simulink library "Near1p1Ann"  (R2022b)
settings: Solver=VariableStepAuto  StartTime=0.0  StopTime=10.0  RelTol=1e-3
libraries: Upmixer1p1Lib x3, FeaturePath x2, FsEQLib x2, HrEQLib x2, Router x2, HandyTextFile x1, TuneVar x1, NearBandSplitLib x1, VolumeMute x1
settings Model: Creator=ak1044356  LastModifiedBy=sa1045272
settings SolverCC: AlgebraicLoopSolver=TrustRegion
settings DebuggingCC: UnconnectedInputMsg=warning  UnconnectedOutputMsg=warning  UnconnectedLineMsg=warning  SFMachineParentedDataDiag=warning  ArithmeticOperatorsInVariantConditions=warning
settings ModelReferenceCC: EnableRefExpFcnMdlSchedulingChecks=on
settings SFSimCC: CustomCodeUndefinedFunction=UseInterfaceOnly

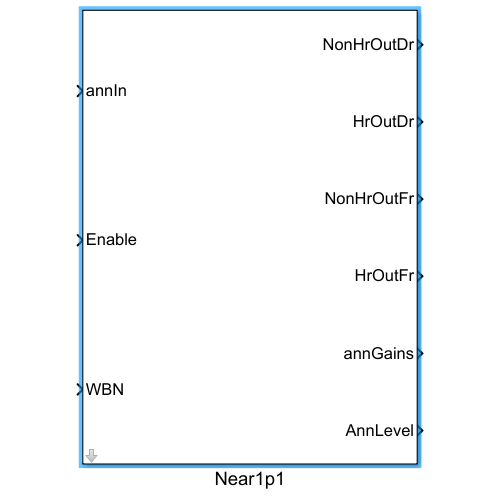
[thumbnail: Simulink's stored preview of the top-level diagram]
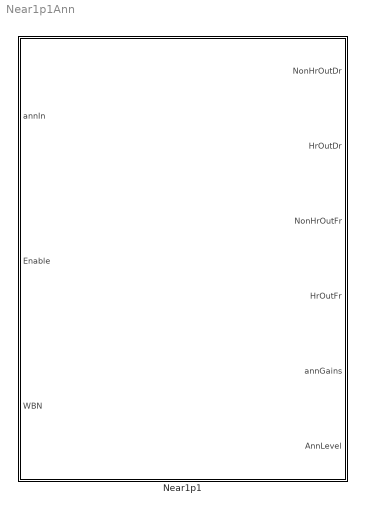
== system Near1p1Ann ==
  Near1p1 : Subsystem  mask{Config=[]}
      mask prompts: Config "Near1p1Config"
      mask init:
      | blkh=gcbh;
      | Config=BTConfig.Assert(blkh,Config);
      | % sample_rate_in_hertz                        = near.sample_rate_in_hertz;
      | % frame_size                                  = near.frame_size;
      | % ann_sysin_channel_count                     = near.ann_sysin_channel_count;
      | % front_peripheral_channel_count              = near.front_peripheral_channel_count;
      | % NEAR1p1FrontPeripheralChannelCountFullRate  = near.NEAR1p1FrontPeripheralChannelCountFullRate;
      | % NearWbAnnCount                              = near.NearWbAnnCount;
      | % headrest_count                              = near.headrest_count;
      | % channels_per_headrest                       = near.channels_per_headrest;
      | % decimation_factor                           = near.decimation_factor;
      | % rear_channel_count                          = near.rear_channel_count;
      | % vm                                          = near.vm;
      | % decimated_frame_size                        = near.decimated_frame_size;
      | % decimated_sample_rate_in_hertz              = near.decimated_sample_rate_in_hertz;
      | Config.Validate();
      | Config.DoMaskInit(blkh);

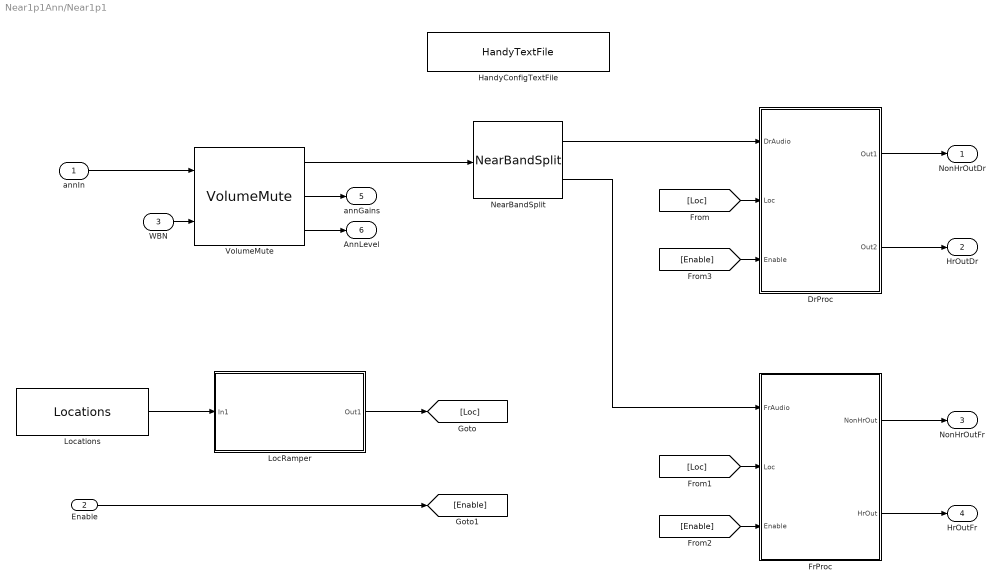
== system Near1p1Ann/Near1p1 ==
  annIn : Inport  OutDataTypeStr=single
  Enable : Inport  Port=2
  WBN : Inport  Port=3
  DrProc : Subsystem
  FrProc : Subsystem
  HandyConfigTextFile : HandyTextFile/HandyTextFile  TemplateSource=Config  FileSuffix=File  OpenDialogOnLoad=off  UseThisBlockName=off  AddGrandParentNamePrefix=off  TheDefaultText=% $(FILENAME) $(PREFIX) $(SUFFIX)  ShowInLibBrowser=on
      settings: SourceProductName=Bose Talaria
  LocRamper : Subsystem
  Locations : Upmixer1p1Lib/Locations  SystemSampleTime=-1  VariantActivationTime=update diagram  Latency=0  AutoFrameSizeCalculation=off
  NearBandSplit : NearBandSplitLib/NearBandSplit  Config=Config.NearBandSplit
  VolumeMute : VolumeMute/VolumeMute  Config=Config.VolumeMute
  NonHrOutDr : Outport  VectorParamsAs1DForOutWhenUnconnected=off
  HrOutDr : Outport  Port=2  VectorParamsAs1DForOutWhenUnconnected=off
  NonHrOutFr : Outport  Port=3  VectorParamsAs1DForOutWhenUnconnected=off
  HrOutFr : Outport  Port=4  VectorParamsAs1DForOutWhenUnconnected=off
  annGains : Outport  Port=5
  AnnLevel : Outport  Port=6
  wires:
  annIn/1 -> VolumeMute/1
  VolumeMute/1 -> NearBandSplit/1
  VolumeMute/2 -> annGains/1
  WBN/1 -> VolumeMute/2
  VolumeMute/3 -> AnnLevel/1
  NearBandSplit/1 -> DrProc/1(DrAudio)
  DrProc/1(Out1) -> NonHrOutDr/1
  DrProc/2(Out2) -> HrOutDr/1
  NearBandSplit/2 -> FrProc/1(FrAudio)
  FrProc/1(NonHrOut) -> NonHrOutFr/1
  FrProc/2(HrOut) -> HrOutFr/1
  Enable/1 -> [Enable]
  Locations/1 -> LocRamper/1(In1)
  [Loc] -> DrProc/2(Loc)
  [Loc] -> FrProc/2(Loc)
  [Enable] -> FrProc/3(Enable)
  [Enable] -> DrProc/3(Enable)
  LocRamper/1(Out1) -> [Loc]

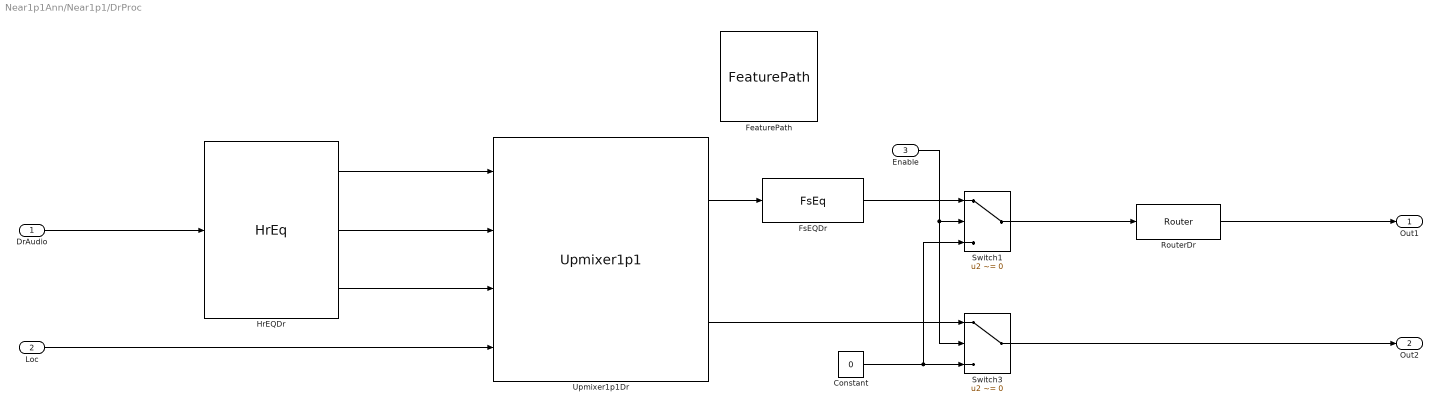
== system Near1p1Ann/Near1p1/DrProc ==
  DrAudio : Inport
  Loc : Inport  Port=2
  Enable : Inport  Port=3
  Constant : Constant  Value=0  OutDataTypeStr=single
  FeaturePath : FeaturePath/FeaturePath  FeatureName=Dr_  IsGroup=off  GroupNumber=-1  IsModule=off  TriggerInit=[730 -106 845 1]
      settings: SourceProductName=Bose Talaria
  FsEQDr : FsEQLib/FsEq  Config=Config.FsEqDr
  HrEQDr : HrEQLib/HrEq  Config=Config.HrEqDr
  RouterDr : Router/Router  nInRouterMask=Config.NearRouterNumIn  nOutRouterMask=Config.NearRouterNumOut  outputMapDefaultRouterMask=Config.NearRouterMap
  Switch1 : Switch  Criteria=u2 ~= 0  Threshold=.5  ZeroCross=off  SaturateOnIntegerOverflow=off  InputSameDT=off
  Switch3 : Switch  Criteria=u2 ~= 0  Threshold=.5  ZeroCross=off  SaturateOnIntegerOverflow=off  InputSameDT=off
  Upmixer1p1Dr : Upmixer1p1Lib/Upmixer1p1  Config=Config.Upmixer1p1Dr
  Out1 : Outport
  Out2 : Outport  Port=2
  wires:
  Switch1/1 -> RouterDr/1
  Constant/1 -> Switch1/3, Switch3/3
  RouterDr/1 -> Out1/1
  FsEQDr/1 -> Switch1/1
  Switch3/1 -> Out2/1
  Enable/1 -> Switch3/2, Switch1/2
  Loc/1 -> Upmixer1p1Dr/4
  DrAudio/1 -> HrEQDr/1
  Upmixer1p1Dr/2 -> Switch3/1
  Upmixer1p1Dr/1 -> FsEQDr/1
  HrEQDr/3 -> Upmixer1p1Dr/3
  HrEQDr/1 -> Upmixer1p1Dr/1
  HrEQDr/2 -> Upmixer1p1Dr/2

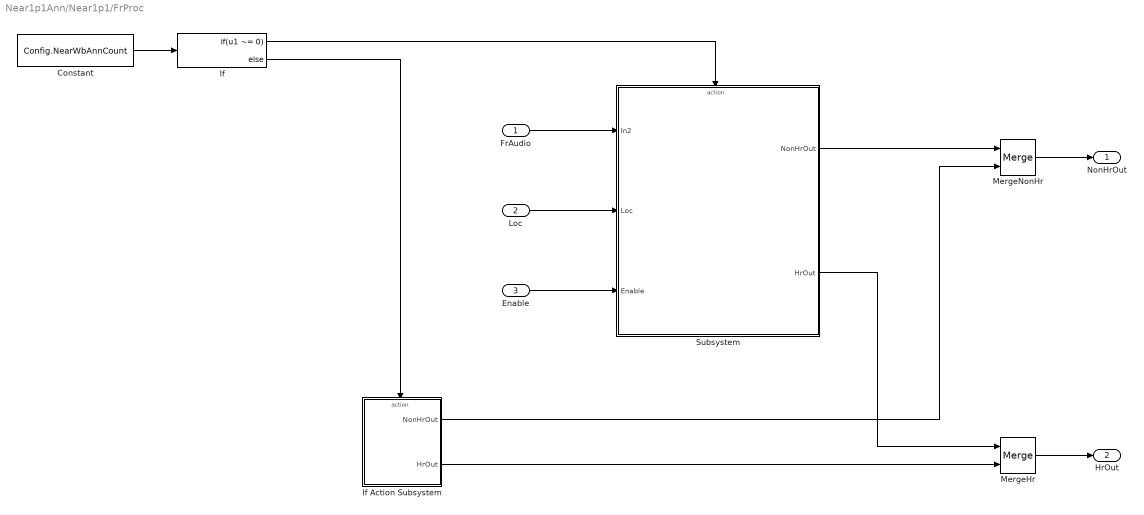
== system Near1p1Ann/Near1p1/FrProc ==
  FrAudio : Inport
  Loc : Inport  Port=2
  Enable : Inport  Port=3
  Constant : Constant  Value=Config.NearWbAnnCount
  If : If  IfExpression=u1 ~= 0
  If Action Subsystem : Subsystem  TreatAsAtomicUnit=on
  MergeHr : Merge
  MergeNonHr : Merge
  Subsystem : Subsystem
  NonHrOut : Outport
  HrOut : Outport  Port=2
  wires:
  Enable/1 -> Subsystem/3(Enable)
  FrAudio/1 -> Subsystem/1(In2)
  Loc/1 -> Subsystem/2(Loc)
  Subsystem/1(NonHrOut) -> MergeNonHr/1
  Subsystem/2(HrOut) -> MergeHr/1
  If/1 -> Subsystem/Action
  If/2 -> If Action Subsystem/Action
  MergeHr/1 -> HrOut/1
  MergeNonHr/1 -> NonHrOut/1
  If Action Subsystem/1(NonHrOut) -> MergeNonHr/2
  If Action Subsystem/2(HrOut) -> MergeHr/2
  Constant/1 -> If/1

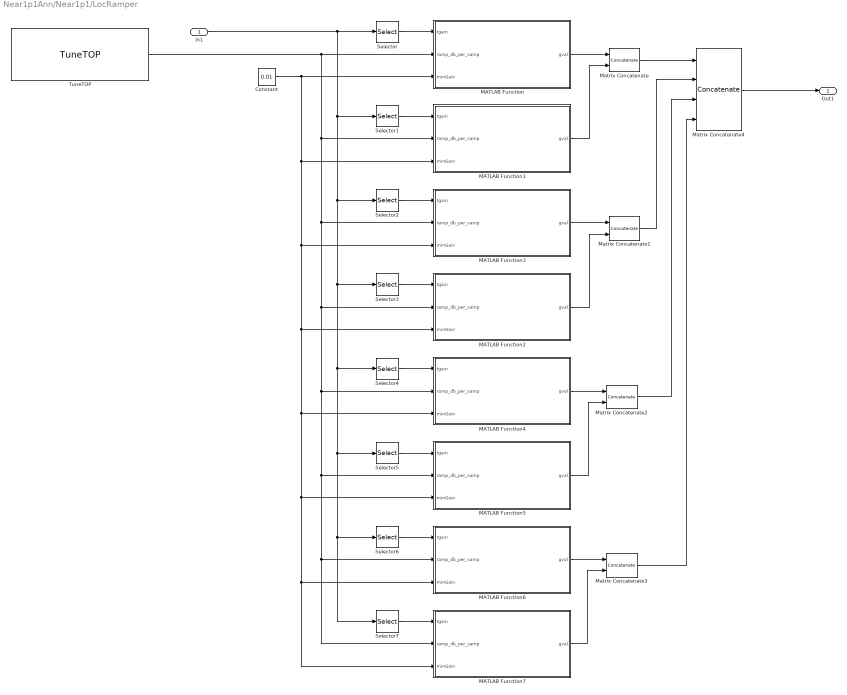
== system Near1p1Ann/Near1p1/LocRamper ==
  In1 : Inport
  Constant : Constant  Value=0.01
  MATLAB Function : MATLAB Function  TreatAsAtomicUnit=on  mask{FRAME_SIZE=Config.FrameSize}
  MATLAB Function1 : MATLAB Function  TreatAsAtomicUnit=on  mask{FRAME_SIZE=Config.FrameSize}
  MATLAB Function2 : MATLAB Function  TreatAsAtomicUnit=on  mask{FRAME_SIZE=Config.FrameSize}
  MATLAB Function3 : MATLAB Function  TreatAsAtomicUnit=on  mask{FRAME_SIZE=Config.FrameSize}
  MATLAB Function4 : MATLAB Function  TreatAsAtomicUnit=on  mask{FRAME_SIZE=Config.FrameSize}
  MATLAB Function5 : MATLAB Function  TreatAsAtomicUnit=on  mask{FRAME_SIZE=Config.FrameSize}
  MATLAB Function6 : MATLAB Function  TreatAsAtomicUnit=on  mask{FRAME_SIZE=Config.FrameSize}
  MATLAB Function7 : MATLAB Function  TreatAsAtomicUnit=on  mask{FRAME_SIZE=Config.FrameSize}
  Matrix Concatenate{,1..3} (4 alike) : Concatenate  Mode=Multidimensional array
  Matrix Concatenate4 : Concatenate  NumInputs=4  Mode=Multidimensional array  ConcatenateDimension=3
  Selector : Selector  NumberOfDimensions=3  InputPortWidth=3  IndexOptions=Index vector (dialog),Index vector (dialog),Index vector (dialog)  Indices=1,1,1  OutputSizes=1,1,1
  Selector1 : Selector  NumberOfDimensions=3  InputPortWidth=3  IndexOptions=Index vector (dialog),Index vector (dialog),Index vector (dialog)  Indices=2,1,1  OutputSizes=1,1,1
  Selector2 : Selector  NumberOfDimensions=3  InputPortWidth=3  IndexOptions=Index vector (dialog),Index vector (dialog),Index vector (dialog)  Indices=1,1,2  OutputSizes=1,1,1
  Selector3 : Selector  NumberOfDimensions=3  InputPortWidth=3  IndexOptions=Index vector (dialog),Index vector (dialog),Index vector (dialog)  Indices=2,1,2  OutputSizes=1,1,1
  Selector4 : Selector  NumberOfDimensions=3  InputPortWidth=3  IndexOptions=Index vector (dialog),Index vector (dialog),Index vector (dialog)  Indices=1,1,3  OutputSizes=1,1,1
  Selector5 : Selector  NumberOfDimensions=3  InputPortWidth=3  IndexOptions=Index vector (dialog),Index vector (dialog),Index vector (dialog)  Indices=2,1,3  OutputSizes=1,1,1
  Selector6 : Selector  NumberOfDimensions=3  InputPortWidth=3  IndexOptions=Index vector (dialog),Index vector (dialog),Index vector (dialog)  Indices=1,1,4  OutputSizes=1,1,1
  Selector7 : Selector  NumberOfDimensions=3  InputPortWidth=3  IndexOptions=Index vector (dialog),Index vector (dialog),Index vector (dialog)  Indices=2,1,4  OutputSizes=1,1,1
  TuneTOP : TuneVar/TuneTOP  TriggerInit=[-300 49 -55 141]  TopName=RampDbPerSample  TuneName=RampDbPerSample  DataType=single  TunabilityNumber=1  MinValue=[]  MaxValue=[]  BankNumber=0  PreOverlay=false  PostOverlay=false  UseSameName=on  MaskValue=Config.DefaultRampDbPerSample
      settings: SourceProductName=Bose Talaria
  Out1 : Outport
  wires:
  Selector/1 -> MATLAB Function/1(tgain)
  TuneTOP/1 -> MATLAB Function7/2(ramp_db_per_samp), MATLAB Function6/2(ramp_db_per_samp), MATLAB Function5/2(ramp_db_per_samp), MATLAB Function4/2(ramp_db_per_samp), MATLAB Function2/2(ramp_db_per_samp), MATLAB Function3/2(ramp_db_per_samp), MATLAB Function1/2(ramp_db_per_samp), MATLAB Function/2(ramp_db_per_samp)
  Matrix Concatenate1/1 -> Matrix Concatenate4/2
  MATLAB Function2/1(gval) -> Matrix Concatenate1/2
  In1/1 -> Selector7/1, Selector6/1, Selector5/1, Selector4/1, Selector3/1, Selector2/1, Selector1/1, Selector/1
  Matrix Concatenate/1 -> Matrix Concatenate4/1
  Selector7/1 -> MATLAB Function7/1(tgain)
  MATLAB Function/1(gval) -> Matrix Concatenate/1
  Selector2/1 -> MATLAB Function3/1(tgain)
  Selector5/1 -> MATLAB Function5/1(tgain)
  MATLAB Function4/1(gval) -> Matrix Concatenate2/1
  Selector1/1 -> MATLAB Function1/1(tgain)
  Selector3/1 -> MATLAB Function2/1(tgain)
  MATLAB Function6/1(gval) -> Matrix Concatenate3/1
  Matrix Concatenate2/1 -> Matrix Concatenate4/3
  MATLAB Function1/1(gval) -> Matrix Concatenate/2
  Selector6/1 -> MATLAB Function6/1(tgain)
  Matrix Concatenate4/1 -> Out1/1
  MATLAB Function7/1(gval) -> Matrix Concatenate3/2
  Matrix Concatenate3/1 -> Matrix Concatenate4/4
  Selector4/1 -> MATLAB Function4/1(tgain)
  MATLAB Function5/1(gval) -> Matrix Concatenate2/2
  MATLAB Function3/1(gval) -> Matrix Concatenate1/1
  Constant/1 -> MATLAB Function7/3(minGain), MATLAB Function6/3(minGain), MATLAB Function5/3(minGain), MATLAB Function4/3(minGain), MATLAB Function2/3(minGain), MATLAB Function3/3(minGain), MATLAB Function1/3(minGain), MATLAB Function/3(minGain)

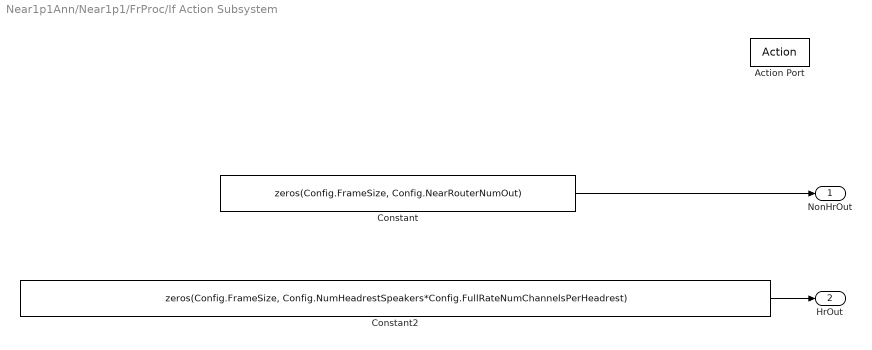
== system Near1p1Ann/Near1p1/FrProc/If Action Subsystem ==
  Action Port : ActionPort  ActionPortLabel=else
  Constant : Constant  Value=zeros(Config.FrameSize, Config.NearRouterNumOut)  OutDataTypeStr=single
  Constant2 : Constant  Value=zeros(Config.FrameSize, Config.NumHeadrestSpeakers*Config.FullRateNumChannelsPerHeadrest)  OutDataTypeStr=single
  NonHrOut : Outport
  HrOut : Outport  Port=2
  wires:
  Constant/1 -> NonHrOut/1
  Constant2/1 -> HrOut/1

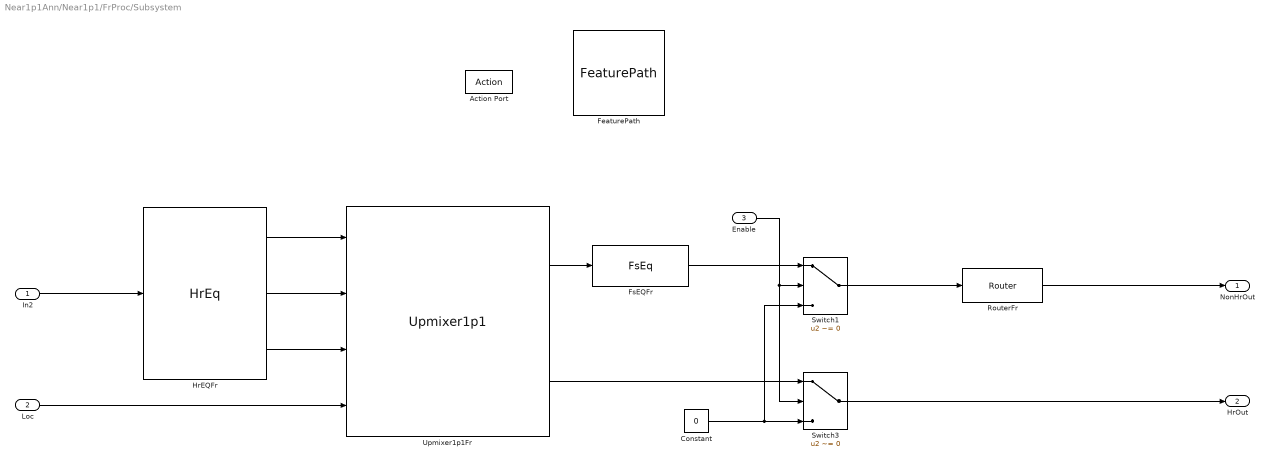
== system Near1p1Ann/Near1p1/FrProc/Subsystem ==
  In2 : Inport
  Loc : Inport  Port=2
  Enable : Inport  Port=3
  Action Port : ActionPort  PropagateVarSize=During execution  ActionPortLabel=if(u1 ~= 0)
  Constant : Constant  Value=0  OutDataTypeStr=single
  FeaturePath : FeaturePath/FeaturePath  FeatureName=Fr_  IsGroup=off  GroupNumber=-1  IsModule=off  TriggerInit=[760 79 875 186]
      settings: SourceProductName=Bose Talaria
  FsEQFr : FsEQLib/FsEq  Config=Config.FsEqFr
  HrEQFr : HrEQLib/HrEq  Config=Config.HrEqFr
  RouterFr : Router/Router  nInRouterMask=Config.NearRouterNumIn  nOutRouterMask=Config.NearRouterNumOut  outputMapDefaultRouterMask=Config.NearRouterMap
  Switch1 : Switch  Criteria=u2 ~= 0  Threshold=.5  ZeroCross=off  SaturateOnIntegerOverflow=off  InputSameDT=off
  Switch3 : Switch  Criteria=u2 ~= 0  Threshold=.5  ZeroCross=off  SaturateOnIntegerOverflow=off  InputSameDT=off
  Upmixer1p1Fr : Upmixer1p1Lib/Upmixer1p1  Config=Config.Upmixer1p1Fr
  NonHrOut : Outport
  HrOut : Outport  Port=2
  wires:
  FsEQFr/1 -> Switch1/1
  Constant/1 -> Switch1/3, Switch3/3
  In2/1 -> HrEQFr/1
  Switch1/1 -> RouterFr/1
  Enable/1 -> Switch3/2, Switch1/2
  RouterFr/1 -> NonHrOut/1
  Switch3/1 -> HrOut/1
  Upmixer1p1Fr/1 -> FsEQFr/1
  Upmixer1p1Fr/2 -> Switch3/1
  Loc/1 -> Upmixer1p1Fr/4
  HrEQFr/3 -> Upmixer1p1Fr/3
  HrEQFr/2 -> Upmixer1p1Fr/2
  HrEQFr/1 -> Upmixer1p1Fr/1

== matlab function Near1p1Ann/Near1p1/LocRamper/MATLAB Function ==
  data: tgain input; gval output; ramp_db_per_samp input; minGain input; FRAME_SIZE parameter
function gval = ramp(tgain, ramp_db_per_samp, minGain, FRAME_SIZE)
% FRAME_SIZE = 32;
% Ramp coefficients
persistent lastTGain;
if (isempty(lastTGain)), lastTGain = cast(tgain + 1, class(tgain)); end
persistent lastG;
if (isempty(lastG)), lastG = cast(0, class(tgain)); end
% Ramp coefficients
persistent upCoeff;
if (isempty(upCoeff)), upCoeff = cast(0, class(tgain)); end
persistent upCoeffN;
if (isempty(upCoeffN)), upCoeffN = cast(0, class(tgain)); end
persistent downCoeff;
if (isempty(downCoeff)), downCoeff = cast(0, class(tgain)); end
persistent downCoeffN;
if (isempty(downCoeffN)), downCoeffN = cast(0, class(tgain)); end
persistent nextUpCoeff;
persistent nextUpCoeffN;
persistent nextDownCoeff;
persistent nextDownCoeffN;
persistent lpfCoeff;
if (isempty(lpfCoeff)), lpfCoeff = cast(exp(-1 / FRAME_SIZE), class(tgain)); end
% Update the next set of ramp coefficients to use
nextUpCoeff = cast(10 ^ abs(ramp_db_per_samp / 20), class(tgain));
nextUpCoeffN = cast(nextUpCoeff ^ FRAME_SIZE, class(tgain));
nextDownCoeff = cast(10 ^ (-abs(ramp_db_per_samp) / 20), class(tgain));
nextDownCoeffN = cast(nextDownCoeff ^ FRAME_SIZE, class(tgain));
% Switch to the next set of ramp coefficients if the target gain changed
chtgain = (tgain ~= lastTGain);
lastTGain = tgain;
if (chtgain)
    upCoeff = nextUpCoeff;
    upCoeffN = nextUpCoeffN;
    downCoeff = nextDownCoeff;
    downCoeffN = nextDownCoeffN;
end
% Initialize output
gp = lastG;
gdiff = tgain - gp;
% By default, use the lpf filter
a = lpfCoeff;
b0 = 1-a;

if (abs(gdiff) < minGain)
    % Snap to target gain if it's close enough
    gVec = tgain * ones(FRAME_SIZE, 1, class(tgain));
else
    if (gdiff > 0)
        % previous gain cannot be zero for exponential ramp
        temp = max(gp, minGain);
        if (temp * upCoeffN < tgain)
            % Ramp not done, so do zero-input exponential ramp
            a = upCoeff;
            b0 = cast(0, class(tgain));
            gp = temp;
        end
    else
        if (gp * downCoeffN > tgain)
            % Ramp not done, so do zero-input exponential ramp
            a = downCoeff;
            b0 = cast(0, class(tgain));
        end
    end
    % Calculate gain
    zi = a * gp;
    gVec = zeros(FRAME_SIZE, 1, class(tgain));
    for samp = 1:FRAME_SIZE
        g = b0 * tgain + zi;
        zi = a * g;
        gVec(samp) = g;
    end
end
lastG = gVec(end);
gval = lastG;
end

== matlab function Near1p1Ann/Near1p1/LocRamper/MATLAB Function1 ==
  data: tgain input; gval output; ramp_db_per_samp input; minGain input; FRAME_SIZE parameter
function gval = ramp(tgain, ramp_db_per_samp, minGain, FRAME_SIZE)
% FRAME_SIZE = 32;
% Ramp coefficients
persistent lastTGain;
if (isempty(lastTGain)), lastTGain = cast(tgain + 1, class(tgain)); end
persistent lastG;
if (isempty(lastG)), lastG = cast(0, class(tgain)); end
% Ramp coefficients
persistent upCoeff;
if (isempty(upCoeff)), upCoeff = cast(0, class(tgain)); end
persistent upCoeffN;
if (isempty(upCoeffN)), upCoeffN = cast(0, class(tgain)); end
persistent downCoeff;
if (isempty(downCoeff)), downCoeff = cast(0, class(tgain)); end
persistent downCoeffN;
if (isempty(downCoeffN)), downCoeffN = cast(0, class(tgain)); end
persistent nextUpCoeff;
persistent nextUpCoeffN;
persistent nextDownCoeff;
persistent nextDownCoeffN;
persistent lpfCoeff;
if (isempty(lpfCoeff)), lpfCoeff = cast(exp(-1 / FRAME_SIZE), class(tgain)); end
% Update the next set of ramp coefficients to use
nextUpCoeff = cast(10 ^ abs(ramp_db_per_samp / 20), class(tgain));
nextUpCoeffN = cast(nextUpCoeff ^ FRAME_SIZE, class(tgain));
nextDownCoeff = cast(10 ^ (-abs(ramp_db_per_samp) / 20), class(tgain));
nextDownCoeffN = cast(nextDownCoeff ^ FRAME_SIZE, class(tgain));
% Switch to the next set of ramp coefficients if the target gain changed
chtgain = (tgain ~= lastTGain);
lastTGain = tgain;
if (chtgain)
    upCoeff = nextUpCoeff;
    upCoeffN = nextUpCoeffN;
    downCoeff = nextDownCoeff;
    downCoeffN = nextDownCoeffN;
end
% Initialize output
gp = lastG;
gdiff = tgain - gp;
% By default, use the lpf filter
a = lpfCoeff;
b0 = 1-a;

if (abs(gdiff) < minGain)
    % Snap to target gain if it's close enough
    gVec = tgain * ones(FRAME_SIZE, 1, class(tgain));
else
    if (gdiff > 0)
        % previous gain cannot be zero for exponential ramp
        temp = max(gp, minGain);
        if (temp * upCoeffN < tgain)
            % Ramp not done, so do zero-input exponential ramp
            a = upCoeff;
            b0 = cast(0, class(tgain));
            gp = temp;
        end
    else
        if (gp * downCoeffN > tgain)
            % Ramp not done, so do zero-input exponential ramp
            a = downCoeff;
            b0 = cast(0, class(tgain));
        end
    end
    % Calculate gain
    zi = a * gp;
    gVec = zeros(FRAME_SIZE, 1, class(tgain));
    for samp = 1:FRAME_SIZE
        g = b0 * tgain + zi;
        zi = a * g;
        gVec(samp) = g;
    end
end
lastG = gVec(end);
gval = lastG;
end

== matlab function Near1p1Ann/Near1p1/LocRamper/MATLAB Function2 ==
  data: tgain input; gval output; ramp_db_per_samp input; minGain input; FRAME_SIZE parameter
function gval = ramp(tgain, ramp_db_per_samp, minGain, FRAME_SIZE)
% FRAME_SIZE = 32;
% Ramp coefficients
persistent lastTGain;
if (isempty(lastTGain)), lastTGain = cast(tgain + 1, class(tgain)); end
persistent lastG;
if (isempty(lastG)), lastG = cast(0, class(tgain)); end
% Ramp coefficients
persistent upCoeff;
if (isempty(upCoeff)), upCoeff = cast(0, class(tgain)); end
persistent upCoeffN;
if (isempty(upCoeffN)), upCoeffN = cast(0, class(tgain)); end
persistent downCoeff;
if (isempty(downCoeff)), downCoeff = cast(0, class(tgain)); end
persistent downCoeffN;
if (isempty(downCoeffN)), downCoeffN = cast(0, class(tgain)); end
persistent nextUpCoeff;
persistent nextUpCoeffN;
persistent nextDownCoeff;
persistent nextDownCoeffN;
persistent lpfCoeff;
if (isempty(lpfCoeff)), lpfCoeff = cast(exp(-1 / FRAME_SIZE), class(tgain)); end
% Update the next set of ramp coefficients to use
nextUpCoeff = cast(10 ^ abs(ramp_db_per_samp / 20), class(tgain));
nextUpCoeffN = cast(nextUpCoeff ^ FRAME_SIZE, class(tgain));
nextDownCoeff = cast(10 ^ (-abs(ramp_db_per_samp) / 20), class(tgain));
nextDownCoeffN = cast(nextDownCoeff ^ FRAME_SIZE, class(tgain));
% Switch to the next set of ramp coefficients if the target gain changed
chtgain = (tgain ~= lastTGain);
lastTGain = tgain;
if (chtgain)
    upCoeff = nextUpCoeff;
    upCoeffN = nextUpCoeffN;
    downCoeff = nextDownCoeff;
    downCoeffN = nextDownCoeffN;
end
% Initialize output
gp = lastG;
gdiff = tgain - gp;
% By default, use the lpf filter
a = lpfCoeff;
b0 = 1-a;

if (abs(gdiff) < minGain)
    % Snap to target gain if it's close enough
    gVec = tgain * ones(FRAME_SIZE, 1, class(tgain));
else
    if (gdiff > 0)
        % previous gain cannot be zero for exponential ramp
        temp = max(gp, minGain);
        if (temp * upCoeffN < tgain)
            % Ramp not done, so do zero-input exponential ramp
            a = upCoeff;
            b0 = cast(0, class(tgain));
            gp = temp;
        end
    else
        if (gp * downCoeffN > tgain)
            % Ramp not done, so do zero-input exponential ramp
            a = downCoeff;
            b0 = cast(0, class(tgain));
        end
    end
    % Calculate gain
    zi = a * gp;
    gVec = zeros(FRAME_SIZE, 1, class(tgain));
    for samp = 1:FRAME_SIZE
        g = b0 * tgain + zi;
        zi = a * g;
        gVec(samp) = g;
    end
end
lastG = gVec(end);
gval = lastG;
end

== matlab function Near1p1Ann/Near1p1/LocRamper/MATLAB Function3 ==
  data: tgain input; gval output; ramp_db_per_samp input; minGain input; FRAME_SIZE parameter
function gval = ramp(tgain, ramp_db_per_samp, minGain, FRAME_SIZE)
% FRAME_SIZE = 32;
% Ramp coefficients
persistent lastTGain;
if (isempty(lastTGain)), lastTGain = cast(tgain + 1, class(tgain)); end
persistent lastG;
if (isempty(lastG)), lastG = cast(0, class(tgain)); end
% Ramp coefficients
persistent upCoeff;
if (isempty(upCoeff)), upCoeff = cast(0, class(tgain)); end
persistent upCoeffN;
if (isempty(upCoeffN)), upCoeffN = cast(0, class(tgain)); end
persistent downCoeff;
if (isempty(downCoeff)), downCoeff = cast(0, class(tgain)); end
persistent downCoeffN;
if (isempty(downCoeffN)), downCoeffN = cast(0, class(tgain)); end
persistent nextUpCoeff;
persistent nextUpCoeffN;
persistent nextDownCoeff;
persistent nextDownCoeffN;
persistent lpfCoeff;
if (isempty(lpfCoeff)), lpfCoeff = cast(exp(-1 / FRAME_SIZE), class(tgain)); end
% Update the next set of ramp coefficients to use
nextUpCoeff = cast(10 ^ abs(ramp_db_per_samp / 20), class(tgain));
nextUpCoeffN = cast(nextUpCoeff ^ FRAME_SIZE, class(tgain));
nextDownCoeff = cast(10 ^ (-abs(ramp_db_per_samp) / 20), class(tgain));
nextDownCoeffN = cast(nextDownCoeff ^ FRAME_SIZE, class(tgain));
% Switch to the next set of ramp coefficients if the target gain changed
chtgain = (tgain ~= lastTGain);
lastTGain = tgain;
if (chtgain)
    upCoeff = nextUpCoeff;
    upCoeffN = nextUpCoeffN;
    downCoeff = nextDownCoeff;
    downCoeffN = nextDownCoeffN;
end
% Initialize output
gp = lastG;
gdiff = tgain - gp;
% By default, use the lpf filter
a = lpfCoeff;
b0 = 1-a;

if (abs(gdiff) < minGain)
    % Snap to target gain if it's close enough
    gVec = tgain * ones(FRAME_SIZE, 1, class(tgain));
else
    if (gdiff > 0)
        % previous gain cannot be zero for exponential ramp
        temp = max(gp, minGain);
        if (temp * upCoeffN < tgain)
            % Ramp not done, so do zero-input exponential ramp
            a = upCoeff;
            b0 = cast(0, class(tgain));
            gp = temp;
        end
    else
        if (gp * downCoeffN > tgain)
            % Ramp not done, so do zero-input exponential ramp
            a = downCoeff;
            b0 = cast(0, class(tgain));
        end
    end
    % Calculate gain
    zi = a * gp;
    gVec = zeros(FRAME_SIZE, 1, class(tgain));
    for samp = 1:FRAME_SIZE
        g = b0 * tgain + zi;
        zi = a * g;
        gVec(samp) = g;
    end
end
lastG = gVec(end);
gval = lastG;
end

== matlab function Near1p1Ann/Near1p1/LocRamper/MATLAB Function4 ==
  data: tgain input; gval output; ramp_db_per_samp input; minGain input; FRAME_SIZE parameter
function gval = ramp(tgain, ramp_db_per_samp, minGain, FRAME_SIZE)
% FRAME_SIZE = 32;
% Ramp coefficients
persistent lastTGain;
if (isempty(lastTGain)), lastTGain = cast(tgain + 1, class(tgain)); end
persistent lastG;
if (isempty(lastG)), lastG = cast(0, class(tgain)); end
% Ramp coefficients
persistent upCoeff;
if (isempty(upCoeff)), upCoeff = cast(0, class(tgain)); end
persistent upCoeffN;
if (isempty(upCoeffN)), upCoeffN = cast(0, class(tgain)); end
persistent downCoeff;
if (isempty(downCoeff)), downCoeff = cast(0, class(tgain)); end
persistent downCoeffN;
if (isempty(downCoeffN)), downCoeffN = cast(0, class(tgain)); end
persistent nextUpCoeff;
persistent nextUpCoeffN;
persistent nextDownCoeff;
persistent nextDownCoeffN;
persistent lpfCoeff;
if (isempty(lpfCoeff)), lpfCoeff = cast(exp(-1 / FRAME_SIZE), class(tgain)); end
% Update the next set of ramp coefficients to use
nextUpCoeff = cast(10 ^ abs(ramp_db_per_samp / 20), class(tgain));
nextUpCoeffN = cast(nextUpCoeff ^ FRAME_SIZE, class(tgain));
nextDownCoeff = cast(10 ^ (-abs(ramp_db_per_samp) / 20), class(tgain));
nextDownCoeffN = cast(nextDownCoeff ^ FRAME_SIZE, class(tgain));
% Switch to the next set of ramp coefficients if the target gain changed
chtgain = (tgain ~= lastTGain);
lastTGain = tgain;
if (chtgain)
    upCoeff = nextUpCoeff;
    upCoeffN = nextUpCoeffN;
    downCoeff = nextDownCoeff;
    downCoeffN = nextDownCoeffN;
end
% Initialize output
gp = lastG;
gdiff = tgain - gp;
% By default, use the lpf filter
a = lpfCoeff;
b0 = 1-a;

if (abs(gdiff) < minGain)
    % Snap to target gain if it's close enough
    gVec = tgain * ones(FRAME_SIZE, 1, class(tgain));
else
    if (gdiff > 0)
        % previous gain cannot be zero for exponential ramp
        temp = max(gp, minGain);
        if (temp * upCoeffN < tgain)
            % Ramp not done, so do zero-input exponential ramp
            a = upCoeff;
            b0 = cast(0, class(tgain));
            gp = temp;
        end
    else
        if (gp * downCoeffN > tgain)
            % Ramp not done, so do zero-input exponential ramp
            a = downCoeff;
            b0 = cast(0, class(tgain));
        end
    end
    % Calculate gain
    zi = a * gp;
    gVec = zeros(FRAME_SIZE, 1, class(tgain));
    for samp = 1:FRAME_SIZE
        g = b0 * tgain + zi;
        zi = a * g;
        gVec(samp) = g;
    end
end
lastG = gVec(end);
gval = lastG;
end

== matlab function Near1p1Ann/Near1p1/LocRamper/MATLAB Function5 ==
  data: tgain input; gval output; ramp_db_per_samp input; minGain input; FRAME_SIZE parameter
function gval = ramp(tgain, ramp_db_per_samp, minGain, FRAME_SIZE)
% FRAME_SIZE = 32;
% Ramp coefficients
persistent lastTGain;
if (isempty(lastTGain)), lastTGain = cast(tgain + 1, class(tgain)); end
persistent lastG;
if (isempty(lastG)), lastG = cast(0, class(tgain)); end
% Ramp coefficients
persistent upCoeff;
if (isempty(upCoeff)), upCoeff = cast(0, class(tgain)); end
persistent upCoeffN;
if (isempty(upCoeffN)), upCoeffN = cast(0, class(tgain)); end
persistent downCoeff;
if (isempty(downCoeff)), downCoeff = cast(0, class(tgain)); end
persistent downCoeffN;
if (isempty(downCoeffN)), downCoeffN = cast(0, class(tgain)); end
persistent nextUpCoeff;
persistent nextUpCoeffN;
persistent nextDownCoeff;
persistent nextDownCoeffN;
persistent lpfCoeff;
if (isempty(lpfCoeff)), lpfCoeff = cast(exp(-1 / FRAME_SIZE), class(tgain)); end
% Update the next set of ramp coefficients to use
nextUpCoeff = cast(10 ^ abs(ramp_db_per_samp / 20), class(tgain));
nextUpCoeffN = cast(nextUpCoeff ^ FRAME_SIZE, class(tgain));
nextDownCoeff = cast(10 ^ (-abs(ramp_db_per_samp) / 20), class(tgain));
nextDownCoeffN = cast(nextDownCoeff ^ FRAME_SIZE, class(tgain));
% Switch to the next set of ramp coefficients if the target gain changed
chtgain = (tgain ~= lastTGain);
lastTGain = tgain;
if (chtgain)
    upCoeff = nextUpCoeff;
    upCoeffN = nextUpCoeffN;
    downCoeff = nextDownCoeff;
    downCoeffN = nextDownCoeffN;
end
% Initialize output
gp = lastG;
gdiff = tgain - gp;
% By default, use the lpf filter
a = lpfCoeff;
b0 = 1-a;

if (abs(gdiff) < minGain)
    % Snap to target gain if it's close enough
    gVec = tgain * ones(FRAME_SIZE, 1, class(tgain));
else
    if (gdiff > 0)
        % previous gain cannot be zero for exponential ramp
        temp = max(gp, minGain);
        if (temp * upCoeffN < tgain)
            % Ramp not done, so do zero-input exponential ramp
            a = upCoeff;
            b0 = cast(0, class(tgain));
            gp = temp;
        end
    else
        if (gp * downCoeffN > tgain)
            % Ramp not done, so do zero-input exponential ramp
            a = downCoeff;
            b0 = cast(0, class(tgain));
        end
    end
    % Calculate gain
    zi = a * gp;
    gVec = zeros(FRAME_SIZE, 1, class(tgain));
    for samp = 1:FRAME_SIZE
        g = b0 * tgain + zi;
        zi = a * g;
        gVec(samp) = g;
    end
end
lastG = gVec(end);
gval = lastG;
end

== matlab function Near1p1Ann/Near1p1/LocRamper/MATLAB Function6 ==
  data: tgain input; gval output; ramp_db_per_samp input; minGain input; FRAME_SIZE parameter
function gval = ramp(tgain, ramp_db_per_samp, minGain, FRAME_SIZE)
% FRAME_SIZE = 32;
% Ramp coefficients
persistent lastTGain;
if (isempty(lastTGain)), lastTGain = cast(tgain + 1, class(tgain)); end
persistent lastG;
if (isempty(lastG)), lastG = cast(0, class(tgain)); end
% Ramp coefficients
persistent upCoeff;
if (isempty(upCoeff)), upCoeff = cast(0, class(tgain)); end
persistent upCoeffN;
if (isempty(upCoeffN)), upCoeffN = cast(0, class(tgain)); end
persistent downCoeff;
if (isempty(downCoeff)), downCoeff = cast(0, class(tgain)); end
persistent downCoeffN;
if (isempty(downCoeffN)), downCoeffN = cast(0, class(tgain)); end
persistent nextUpCoeff;
persistent nextUpCoeffN;
persistent nextDownCoeff;
persistent nextDownCoeffN;
persistent lpfCoeff;
if (isempty(lpfCoeff)), lpfCoeff = cast(exp(-1 / FRAME_SIZE), class(tgain)); end
% Update the next set of ramp coefficients to use
nextUpCoeff = cast(10 ^ abs(ramp_db_per_samp / 20), class(tgain));
nextUpCoeffN = cast(nextUpCoeff ^ FRAME_SIZE, class(tgain));
nextDownCoeff = cast(10 ^ (-abs(ramp_db_per_samp) / 20), class(tgain));
nextDownCoeffN = cast(nextDownCoeff ^ FRAME_SIZE, class(tgain));
% Switch to the next set of ramp coefficients if the target gain changed
chtgain = (tgain ~= lastTGain);
lastTGain = tgain;
if (chtgain)
    upCoeff = nextUpCoeff;
    upCoeffN = nextUpCoeffN;
    downCoeff = nextDownCoeff;
    downCoeffN = nextDownCoeffN;
end
% Initialize output
gp = lastG;
gdiff = tgain - gp;
% By default, use the lpf filter
a = lpfCoeff;
b0 = 1-a;

if (abs(gdiff) < minGain)
    % Snap to target gain if it's close enough
    gVec = tgain * ones(FRAME_SIZE, 1, class(tgain));
else
    if (gdiff > 0)
        % previous gain cannot be zero for exponential ramp
        temp = max(gp, minGain);
        if (temp * upCoeffN < tgain)
            % Ramp not done, so do zero-input exponential ramp
            a = upCoeff;
            b0 = cast(0, class(tgain));
            gp = temp;
        end
    else
        if (gp * downCoeffN > tgain)
            % Ramp not done, so do zero-input exponential ramp
            a = downCoeff;
            b0 = cast(0, class(tgain));
        end
    end
    % Calculate gain
    zi = a * gp;
    gVec = zeros(FRAME_SIZE, 1, class(tgain));
    for samp = 1:FRAME_SIZE
        g = b0 * tgain + zi;
        zi = a * g;
        gVec(samp) = g;
    end
end
lastG = gVec(end);
gval = lastG;
end

== matlab function Near1p1Ann/Near1p1/LocRamper/MATLAB Function7 ==
  data: tgain input; gval output; ramp_db_per_samp input; minGain input; FRAME_SIZE parameter
function gval = ramp(tgain, ramp_db_per_samp, minGain, FRAME_SIZE)
% FRAME_SIZE = 32;
% Ramp coefficients
persistent lastTGain;
if (isempty(lastTGain)), lastTGain = cast(tgain + 1, class(tgain)); end
persistent lastG;
if (isempty(lastG)), lastG = cast(0, class(tgain)); end
% Ramp coefficients
persistent upCoeff;
if (isempty(upCoeff)), upCoeff = cast(0, class(tgain)); end
persistent upCoeffN;
if (isempty(upCoeffN)), upCoeffN = cast(0, class(tgain)); end
persistent downCoeff;
if (isempty(downCoeff)), downCoeff = cast(0, class(tgain)); end
persistent downCoeffN;
if (isempty(downCoeffN)), downCoeffN = cast(0, class(tgain)); end
persistent nextUpCoeff;
persistent nextUpCoeffN;
persistent nextDownCoeff;
persistent nextDownCoeffN;
persistent lpfCoeff;
if (isempty(lpfCoeff)), lpfCoeff = cast(exp(-1 / FRAME_SIZE), class(tgain)); end
% Update the next set of ramp coefficients to use
nextUpCoeff = cast(10 ^ abs(ramp_db_per_samp / 20), class(tgain));
nextUpCoeffN = cast(nextUpCoeff ^ FRAME_SIZE, class(tgain));
nextDownCoeff = cast(10 ^ (-abs(ramp_db_per_samp) / 20), class(tgain));
nextDownCoeffN = cast(nextDownCoeff ^ FRAME_SIZE, class(tgain));
% Switch to the next set of ramp coefficients if the target gain changed
chtgain = (tgain ~= lastTGain);
lastTGain = tgain;
if (chtgain)
    upCoeff = nextUpCoeff;
    upCoeffN = nextUpCoeffN;
    downCoeff = nextDownCoeff;
    downCoeffN = nextDownCoeffN;
end
% Initialize output
gp = lastG;
gdiff = tgain - gp;
% By default, use the lpf filter
a = lpfCoeff;
b0 = 1-a;

if (abs(gdiff) < minGain)
    % Snap to target gain if it's close enough
    gVec = tgain * ones(FRAME_SIZE, 1, class(tgain));
else
    if (gdiff > 0)
        % previous gain cannot be zero for exponential ramp
        temp = max(gp, minGain);
        if (temp * upCoeffN < tgain)
            % Ramp not done, so do zero-input exponential ramp
            a = upCoeff;
            b0 = cast(0, class(tgain));
            gp = temp;
        end
    else
        if (gp * downCoeffN > tgain)
            % Ramp not done, so do zero-input exponential ramp
            a = downCoeff;
            b0 = cast(0, class(tgain));
        end
    end
    % Calculate gain
    zi = a * gp;
    gVec = zeros(FRAME_SIZE, 1, class(tgain));
    for samp = 1:FRAME_SIZE
        g = b0 * tgain + zi;
        zi = a * g;
        gVec(samp) = g;
    end
end
lastG = gVec(end);
gval = lastG;
end
